simulink model "untitled1"  (R2020b)
settings: Solver=VariableStepAuto  StartTime=0.0  StopTime=10.0  RelTol=1e-3
values from neighbouring files (symbols this model uses):
  b = 50.0    [data.sldd]
  ki = 40.0    [data.sldd]
  kp = 800.0    [data.sldd]
  m = 1000.0    [data.sldd]
settings Model: DataDictionary=data.sldd  Creator=ANUJA  LastModifiedBy=ANUJA

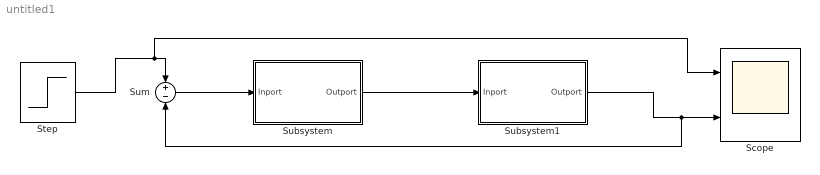
== system untitled1 ==
  Scope : Scope  NumInputPorts=2
  Step : Step  SampleTime=0
  Subsystem : Subsystem
  Subsystem1 : Subsystem
  Sum : Sum  Inputs=+-
  wires:
  Subsystem/1(Outport) -> Subsystem1/1(Inport)
  Step/1 -> Scope/1, Sum/1
  Subsystem1/1(Outport) -> Sum/2, Scope/2
  Sum/1 -> Subsystem/1(Inport)

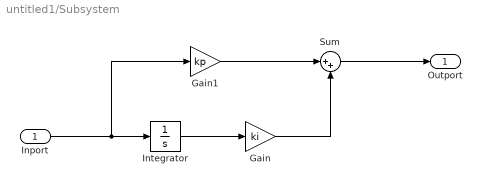
== system untitled1/Subsystem ==
  Inport : Inport  OutDataTypeStr=double  PortDimensions=1  SampleTime=0
  Gain : Gain  Gain=ki
  Gain1 : Gain  Gain=kp
  Integrator : Integrator
  Sum : Sum  Inputs=|++
  Outport : Outport  OutDataTypeStr=double  PortDimensions=1  SampleTime=0
  wires:
  Gain/1 -> Sum/2
  Sum/1 -> Outport/1
  Inport/1 -> Integrator/1, Gain1/1
  Gain1/1 -> Sum/1
  Integrator/1 -> Gain/1

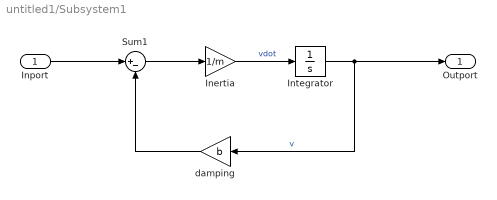
== system untitled1/Subsystem1 ==
  Inport : Inport  OutDataTypeStr=double  PortDimensions=1  SampleTime=0
  Inertia : Gain  Gain=1/m
  Integrator : Integrator
  Sum1 : Sum  Inputs=|+-
  damping : Gain  Gain=b
  Outport : Outport  OutDataTypeStr=double  PortDimensions=1  SampleTime=0
  wires:
  Integrator/1 -> Outport/1, damping/1  "v"
  Sum1/1 -> Inertia/1
  damping/1 -> Sum1/2
  Inport/1 -> Sum1/1
  Inertia/1 -> Integrator/1  "vdot"
